simulink model "pfbfirr_core"  (Simulink 7.9)
settings: Solver=ode45  StartTime=0.0  StopTime=10.0  RelTol=1e-3
undefined symbols (not defined in the file or in its folder): pfb_coeff_gen_calc
libraries: xbsIndex_r4 x844, casper_library_delays x48, casper_library_pfbs x2
(part 1 of 10)
settings Model: Creator=chenhong  LastModifiedBy=ptcs

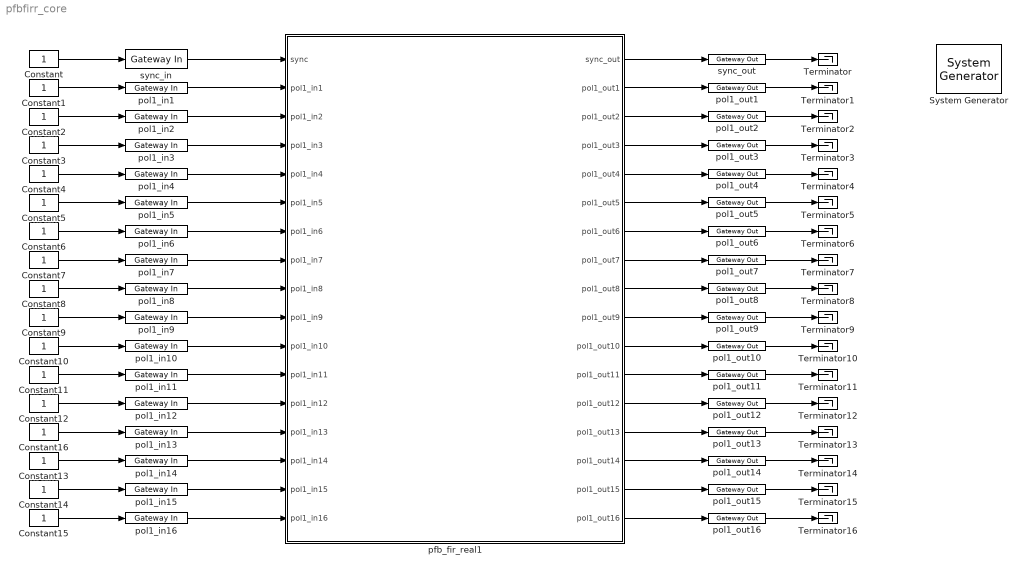
== system pfbfirr_core ==
  " System Generator" : xbsIndex_r4/ System Generator  Tag=genX  xilinxfamily=virtex6  part=xc6vsx475t  speed=-1  package=ff1759  synthesis_tool=XST  clock_wrapper=Clock Enables  directory=./pfbfirr_core  proj_type=Project Navigator  Synth_file=XST Defaults  Impl_file=ISE Defaults  testbench=off  simulink_period=1  sysclk_period=6.6667  dcm_input_clock_period=100  incr_netlist=off  trim_vbits=Everywhere in SubSystem  dbl_ovrd=According to Block Masks  core_generation=According to Block Masks  run_coregen=off  deprecated_control=off  eval_field=0  block_type=sysgen
      settings: block_version=10.1.3
  Constant{,1..16} (17 alike) : Constant
  Terminator{,1..16} (17 alike) : Terminator
  pfb_fir_real1 : Subsystem  AncestorBlock=casper_library_pfbs/pfb_fir_real  mask(pfb_fir_real){PFBSize=15, TotalTaps=4, WindowType=hamming, n_inputs=4, MakeBiplex=off, BitWidthIn=8, BitWidthOut=18, CoeffBitWidth=18, CoeffDistMem=off, add_latency=1, mult_latency=2, bram_latency=2, fan_latency=1, conv_latency=1, quantization=Round  (unbiased: Even Values), fwidth=1, mult_spec=2, adder_folding=on, adder_imp=Fabric, coeffs_share=on}
      mask prompts: PFBSize "Size of PFB: (2^? pnts)"; TotalTaps "Total Number of Taps:"; WindowType "Windowing Function:"; n_inputs "Number of Simultaneous Inputs: (2^?)"; MakeBiplex "Make Biplex?"; BitWidthIn "Input Bitwidth:"; BitWidthOut "Output Bitwidth:"; CoeffBitWidth "Coefficient Bitwidth:"; CoeffDistMem "Use Distributed Memory for Coeffs"; add_latency "Add Latency"; mult_latency "Mult Latency"; bram_latency "BRAM Latency"; fan_latency "Fanout latency"; conv_latency "Convert latency"; quantization "Quantization Behavior"; fwidth "Bin Width Scaling (normal=1)"; mult_spec "Multiplier specification (0=core, 1=embedded, 2=behavioural) (left=1st tap, or just one value)"; adder_folding "Fold adders into DSPs"; adder_imp "Adder implementation"; coeffs_share "Share coefficients between polarisations (use less BRAM)?"
      mask help:
      | Fold adders into DSPs: Causes adders to be absorbed into DSP blocks (supported in Virtex5)
      | Adder implementation: Cores using Fabric or DSP48 or behavioral HDL
      mask init:
      | pfb_fir_real_init(gcb, ...
      |     'PFBSize', PFBSize, ...
      |     'TotalTaps', TotalTaps, ...
      |     'WindowType', WindowType, ...
      |     'n_inputs', n_inputs, ...
      |     'MakeBiplex', MakeBiplex, ...
      |     'BitWidthIn', BitWidthIn, ...
      |     'BitWidthOut', BitWidthOut, ...
      |     'CoeffBitWidth', CoeffBitWidth, ...
      |     'CoeffDistMem', CoeffDistMem, ...
      |     'add_latency', add_latency, ...
      |     'mult_latency', mult_latency, ...
      |     'bram_latency', bram_latency, ...
      |     'fan_latency', fan_latency, ...
      |     'conv_latency', conv_latency, ...
      |     'quantization', quantization, ...
      |     'fwidth', fwidth, ...
      |     'mult_spec', mult_spec, ...
      |     'adder_folding', adder_folding, ...
      |     'adder_imp', adder_imp, ...
      |     'coeffs_share', coeffs_share);
      settings: AttributesFormatString=taps=4, add_latency=1
      mask Help: eval('xlWeb(''http://casper.berkeley.edu/wiki/Pfb_fir_real'')')
      mask StyleString: edit,edit,popup(bartlett|barthannwin|blackman|blackmanharris|bohamwin|chebwin|flattopwin|gausswin|hamming|hann|kaiser|nuttallwin|parzenwin|rectwin|tukeywin|triang|userwindow),edit,checkbox,edit,edit,edit,checkbox,edit,edit,edit,edit,edit,popup(Truncate|Round  (unbiased: +/- Inf)|Round  (unbiased: Even Values)),edit,edit,checkbox,popup(Behavioral|Fabric|DSP48),checkbox
      mask CallbackString:
      | |%num_taps = eval(get_param(gcb, 'TotalTaps'));
      | %old_vec = eval(get_param(gcb, 'mult_spec'));=-0l
      | 
      | %vec = 2.*ones(1,num_taps);
      | %old_size = length(old_vec);
      | 
      | %if(old_size <= num_taps),
      | %    new_size = old_size;
      | %else,
      | %    new_size = num_taps;
      | %end
      | 
      | %for n = 1:new_size, vec(n) = old_vec(n); end
      | %set_param(gcb, 'mult_spec', mat2str(vec));||||||||||||||||||
  pol1_in{1..16} (16 alike) : xbsIndex_r4/Gateway In  gui_display_data_type=Fixed-point  arith_type="Signed  (2's comp)"  n_bits=8  bin_pt=7  preci_type=Single  exp_width=8  frac_width=24  quantization="Round  (unbiased: +/- Inf)"  overflow=Saturate  period=1  dbl_ovrd=off  timing_constraint=None  locs_specified=off  LOCs={}  UseAsADC=off  ADCChannel='1'  inherit_from_input=off  hdl_port=on  block_type=gatewayin
  pol1_out{1..16} (16 alike) : xbsIndex_r4/Gateway Out  inherit_from_input=off  hdl_port=on  timing_constraint=None  locs_specified=off  LOCs={}  UseAsDAC=off  DACChannel='1'  block_type=gatewayout
  sync_in : xbsIndex_r4/Gateway In  gui_display_data_type=Boolean  arith_type=Boolean  n_bits=16  bin_pt=14  preci_type=Single  exp_width=8  frac_width=24  quantization="Round  (unbiased: +/- Inf)"  overflow=Saturate  period=1  dbl_ovrd=off  timing_constraint=None  locs_specified=off  LOCs={}  UseAsADC=off  ADCChannel='1'  inherit_from_input=off  hdl_port=on  block_type=gatewayin
  sync_out : xbsIndex_r4/Gateway Out  inherit_from_input=off  hdl_port=on  timing_constraint=None  locs_specified=off  LOCs={}  UseAsDAC=off  DACChannel='1'  block_type=gatewayout
  wires:
  sync_in/1 -> pfb_fir_real1/1(sync)
  pol1_in1/1 -> pfb_fir_real1/2(pol1_in1)
  pol1_in2/1 -> pfb_fir_real1/3(pol1_in2)
  pol1_in3/1 -> pfb_fir_real1/4(pol1_in3)
  pol1_in4/1 -> pfb_fir_real1/5(pol1_in4)
  pol1_in5/1 -> pfb_fir_real1/6(pol1_in5)
  pol1_in6/1 -> pfb_fir_real1/7(pol1_in6)
  pol1_in7/1 -> pfb_fir_real1/8(pol1_in7)
  pol1_in8/1 -> pfb_fir_real1/9(pol1_in8)
  pol1_in9/1 -> pfb_fir_real1/10(pol1_in9)
  pol1_in10/1 -> pfb_fir_real1/11(pol1_in10)
  pol1_in11/1 -> pfb_fir_real1/12(pol1_in11)
  pol1_in12/1 -> pfb_fir_real1/13(pol1_in12)
  pol1_in13/1 -> pfb_fir_real1/14(pol1_in13)
  pol1_in14/1 -> pfb_fir_real1/15(pol1_in14)
  pol1_in15/1 -> pfb_fir_real1/16(pol1_in15)
  pol1_in16/1 -> pfb_fir_real1/17(pol1_in16)
  pfb_fir_real1/2(pol1_out1) -> pol1_out1/1
  pfb_fir_real1/1(sync_out) -> sync_out/1
  pfb_fir_real1/3(pol1_out2) -> pol1_out2/1
  pfb_fir_real1/4(pol1_out3) -> pol1_out3/1
  pfb_fir_real1/5(pol1_out4) -> pol1_out4/1
  pfb_fir_real1/6(pol1_out5) -> pol1_out5/1
  pfb_fir_real1/7(pol1_out6) -> pol1_out6/1
  pfb_fir_real1/8(pol1_out7) -> pol1_out7/1
  pfb_fir_real1/9(pol1_out8) -> pol1_out8/1
  pfb_fir_real1/10(pol1_out9) -> pol1_out9/1
  pfb_fir_real1/11(pol1_out10) -> pol1_out10/1
  pfb_fir_real1/12(pol1_out11) -> pol1_out11/1
  pfb_fir_real1/13(pol1_out12) -> pol1_out12/1
  pfb_fir_real1/14(pol1_out13) -> pol1_out13/1
  pfb_fir_real1/15(pol1_out14) -> pol1_out14/1
  pfb_fir_real1/16(pol1_out15) -> pol1_out15/1
  pfb_fir_real1/17(pol1_out16) -> pol1_out16/1
  Constant/1 -> sync_in/1
  Constant1/1 -> pol1_in1/1
  Constant2/1 -> pol1_in2/1
  Constant3/1 -> pol1_in3/1
  Constant4/1 -> pol1_in4/1
  Constant5/1 -> pol1_in5/1
  Constant6/1 -> pol1_in6/1
  Constant7/1 -> pol1_in7/1
  Constant8/1 -> pol1_in8/1
  Constant9/1 -> pol1_in9/1
  Constant10/1 -> pol1_in10/1
  Constant11/1 -> pol1_in11/1
  Constant12/1 -> pol1_in12/1
  Constant16/1 -> pol1_in13/1
  Constant13/1 -> pol1_in14/1
  Constant14/1 -> pol1_in15/1
  Constant15/1 -> pol1_in16/1
  sync_out/1 -> Terminator/1
  pol1_out1/1 -> Terminator1/1
  pol1_out2/1 -> Terminator2/1
  pol1_out3/1 -> Terminator3/1
  pol1_out4/1 -> Terminator4/1
  pol1_out5/1 -> Terminator5/1
  pol1_out6/1 -> Terminator6/1
  pol1_out7/1 -> Terminator7/1
  pol1_out8/1 -> Terminator8/1
  pol1_out9/1 -> Terminator9/1
  pol1_out10/1 -> Terminator10/1
  pol1_out11/1 -> Terminator11/1
  pol1_out12/1 -> Terminator12/1
  pol1_out13/1 -> Terminator13/1
  pol1_out14/1 -> Terminator14/1
  pol1_out15/1 -> Terminator15/1
  pol1_out16/1 -> Terminator16/1
